simulink model "ExoSense_v2"  (R2016a)
settings: Solver=FixedStepDiscrete  StartTime=0.0  StopTime=inf  FixedStep=0.2  RelTol=1e-3
libraries: ExoSense_library x5, QB_pacer_lib x1, qbmove_library x1
settings Model: Creator=laurentio  LastModifiedBy=MattiaCP
settings DataIOCC: LimitDataPoints=on  SaveFormat=Array
settings DebuggingCC: UnderspecifiedInitializationDetection=Classic  MergeDetectMultiDrivingBlocksExec=none  SolverPrmCheckMsg=warning  AllowSymbolicDim=off  StateNameClashWarn=warning
settings HardwareCC: ProdBitPerPointer=32  ProdLargestAtomicFloat=None  ProdIntDivRoundTo=Undefined  ProdEndianess=Unspecified  ProdWordSize=32  ProdHWDeviceType=32-bit Generic
settings ModelReferenceCC: PropagateSignalLabelsOutOfModel=off
settings ConfigComp: CovModelRefEnable=Off  CovSFcnEnable=off

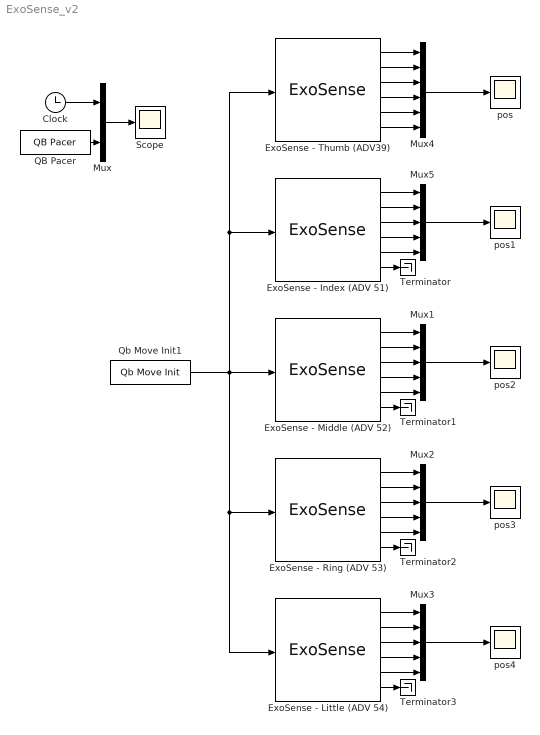
== system ExoSense_v2 ==
  Clock : Clock
  ExoSense - Index (ADV 51) : ExoSense_library/ExoSense  ID=2  ACTIVE_COMM_DIRECTIONS=Rx  CONTROL_MODE=Prime Movers Positions  DAISY_CHAINING=off  MAX_ANG=0  SW_LIMIT=inf  OFFSET=0  ACTIVATE=off  WDT=0.0  UNITY=Degrees
  ExoSense - Little (ADV 54) : ExoSense_library/ExoSense  ID=5  ACTIVE_COMM_DIRECTIONS=Rx  CONTROL_MODE=Prime Movers Positions  DAISY_CHAINING=off  MAX_ANG=0  SW_LIMIT=inf  OFFSET=0  ACTIVATE=off  WDT=0.0  UNITY=Degrees
  ExoSense - Middle (ADV 52) : ExoSense_library/ExoSense  ID=3  ACTIVE_COMM_DIRECTIONS=Rx  CONTROL_MODE=Prime Movers Positions  DAISY_CHAINING=off  MAX_ANG=0  SW_LIMIT=inf  OFFSET=0  ACTIVATE=off  WDT=0.0  UNITY=Degrees
  ExoSense - Ring (ADV 53) : ExoSense_library/ExoSense  ID=4  ACTIVE_COMM_DIRECTIONS=Rx  CONTROL_MODE=Prime Movers Positions  DAISY_CHAINING=off  MAX_ANG=0  SW_LIMIT=inf  OFFSET=0  ACTIVATE=off  WDT=0.0  UNITY=Degrees
  ExoSense - Thumb (ADV39) : ExoSense_library/ExoSense  ID=1  ACTIVE_COMM_DIRECTIONS=Rx  CONTROL_MODE=Prime Movers Positions  DAISY_CHAINING=off  MAX_ANG=0  SW_LIMIT=inf  OFFSET=0  ACTIVATE=off  WDT=0.0  UNITY=Degrees
  Mux : Mux  Inputs=2
  Mux{1..3,5} (4 alike) : Mux  Inputs=5
  Mux4 : Mux  Inputs=6
  QB Pacer : QB_pacer_lib/QB Pacer  simTimePerRealTime=1
  Qb Move Init1 : qbmove_library/Qb Move Init  NUMBER_OF_COM='COM5'  BAUD_RATE_COM=2000000
  Scope : Scope
  Terminator{,1..3} (4 alike) : Terminator
  pos{,1..4} (5 alike) : Scope
  wires:
  Qb Move Init1/1 -> ExoSense - Middle (ADV 52)/1, ExoSense - Little (ADV 54)/1, ExoSense - Ring (ADV 53)/1, ExoSense - Index (ADV 51)/1, ExoSense - Thumb (ADV39)/1
  QB Pacer/1 -> Mux/2
  Clock/1 -> Mux/1
  Mux/1 -> Scope/1
  Mux4/1 -> pos/1
  ExoSense - Thumb (ADV39)/4 -> Mux4/4
  ExoSense - Thumb (ADV39)/3 -> Mux4/3
  ExoSense - Thumb (ADV39)/6 -> Mux4/6
  ExoSense - Thumb (ADV39)/5 -> Mux4/5
  Mux5/1 -> pos1/1
  ExoSense - Index (ADV 51)/2 -> Mux5/2
  ExoSense - Index (ADV 51)/4 -> Mux5/4
  ExoSense - Index (ADV 51)/3 -> Mux5/3
  ExoSense - Index (ADV 51)/6 -> Terminator/1
  ExoSense - Index (ADV 51)/1 -> Mux5/1
  ExoSense - Index (ADV 51)/5 -> Mux5/5
  ExoSense - Thumb (ADV39)/1 -> Mux4/1
  ExoSense - Thumb (ADV39)/2 -> Mux4/2
  Mux1/1 -> pos2/1
  ExoSense - Middle (ADV 52)/2 -> Mux1/2
  ExoSense - Middle (ADV 52)/4 -> Mux1/4
  ExoSense - Middle (ADV 52)/3 -> Mux1/3
  ExoSense - Middle (ADV 52)/6 -> Terminator1/1
  ExoSense - Middle (ADV 52)/1 -> Mux1/1
  ExoSense - Middle (ADV 52)/5 -> Mux1/5
  Mux2/1 -> pos3/1
  ExoSense - Ring (ADV 53)/1 -> Mux2/1
  ExoSense - Ring (ADV 53)/2 -> Mux2/2
  ExoSense - Ring (ADV 53)/3 -> Mux2/3
  ExoSense - Ring (ADV 53)/4 -> Mux2/4
  ExoSense - Ring (ADV 53)/5 -> Mux2/5
  ExoSense - Ring (ADV 53)/6 -> Terminator2/1
  Mux3/1 -> pos4/1
  ExoSense - Little (ADV 54)/1 -> Mux3/1
  ExoSense - Little (ADV 54)/2 -> Mux3/2
  ExoSense - Little (ADV 54)/3 -> Mux3/3
  ExoSense - Little (ADV 54)/4 -> Mux3/4
  ExoSense - Little (ADV 54)/5 -> Mux3/5
  ExoSense - Little (ADV 54)/6 -> Terminator3/1
